simulink model "Hystersis_Relay_Logic"  (R2017a)
settings: Solver=FixedStepDiscrete  StartTime=0.0  StopTime=10.0  FixedStep=0.01  RelTol=1e-3
libraries: simulink x1, simulink_extras x1
settings Model: Creator=ACER  LastModifiedBy=peram
settings DataIOCC: ReturnWorkspaceOutputs=on
settings DebuggingCC: UnconnectedInputMsg=none  UnconnectedOutputMsg=none  UnconnectedLineMsg=none  SFMachineParentedDataDiag=error
settings ModelReferenceCC: EnableRefExpFcnMdlSchedulingChecks=off
settings SFSimCC: SimUseLocalCustomCode=on
settings RTWCC: RTWUseLocalCustomCode=on

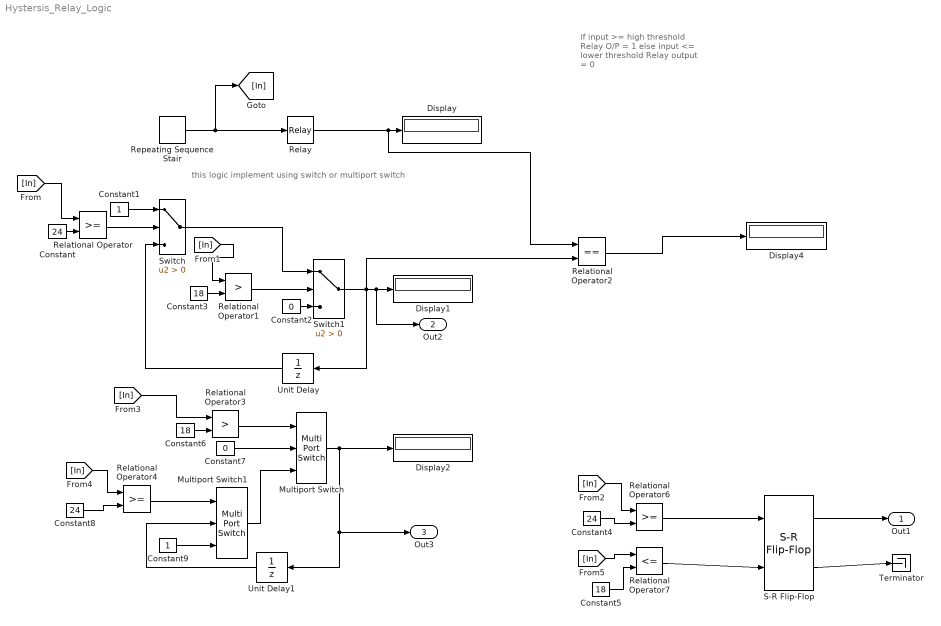
== system Hystersis_Relay_Logic ==
  note: if input >= high threshold
      | Relay O/P = 1
      | else
      | input <= lower threshold
      | Relay output = 0
  note: this logic implement using switch or multiport switch
  Constant : Constant  Value=24  OutDataTypeStr=Inherit: Inherit via back propagation
  Constant1 : Constant
  Constant2 : Constant  Value=0
  Constant3 : Constant  Value=18
  Constant4 : Constant  Value=24
  Constant5 : Constant  Value=18
  Constant6 : Constant  Value=18  OutDataTypeStr=Inherit: Inherit via back propagation
  Constant7 : Constant  Value=0  OutDataTypeStr=Inherit: Inherit via back propagation
  Constant8 : Constant  Value=24  OutDataTypeStr=Inherit: Inherit via back propagation
  Constant9 : Constant  OutDataTypeStr=Inherit: Inherit via back propagation
  Display{,1..2,4} (4 alike) : Display
  Multiport Switch : MultiPortSwitch  DataPortOrder=Zero-based contiguous  Inputs=2  OutDataTypeStr=Inherit: Inherit via back propagation
  Multiport Switch1 : MultiPortSwitch  DataPortOrder=Zero-based contiguous  Inputs=2  OutDataTypeStr=Inherit: Inherit via back propagation
  Relational Operator : RelationalOperator  OutDataTypeStr=boolean  RndMeth=Simplest
  Relational Operator1 : RelationalOperator  Operator=>  OutDataTypeStr=boolean  RndMeth=Simplest
  Relational Operator2 : RelationalOperator  Operator===  OutDataTypeStr=boolean  RndMeth=Simplest
  Relational Operator3 : RelationalOperator  Operator=>  OutDataTypeStr=boolean  RndMeth=Simplest
  Relational Operator4 : RelationalOperator  OutDataTypeStr=boolean  RndMeth=Simplest
  Relational Operator6 : RelationalOperator  OutDataTypeStr=boolean  RndMeth=Simplest
  Relational Operator7 : RelationalOperator  Operator=<=  OutDataTypeStr=boolean  RndMeth=Simplest
  Relay : Relay  OnSwitchValue=24  OffSwitchValue=18
  Repeating Sequence Stair : simulink/Sources/Repeating Sequence Stair  OutValues=[17 18 20 24 27 22 18 17 26 15].'  tsamp=-1  OutMin=[]  OutMax=[]  OutDataTypeStr=uint8  OutputDataTypeScalingMode=uint8  OutDataType=fixdt(0,8)  ConRadixGroup=Best Precision: Vector-wise  OutScaling=2^-12
  S-R Flip-Flop : simulink_extras/Flip Flops/S-R Flip-Flop  initial_condition=0
  Switch : Switch  Criteria=u2 > Threshold  OutDataTypeStr=Inherit: Inherit via back propagation
  Switch1 : Switch  Criteria=u2 > Threshold  OutDataTypeStr=Inherit: Inherit via back propagation
  Terminator : Terminator
  Unit Delay : UnitDelay  SampleTime=-1
  Unit Delay1 : UnitDelay  SampleTime=-1
  Out1 : Outport
  Out2 : Outport  Port=2  OutDataTypeStr=int8
  Out3 : Outport  Port=3  OutDataTypeStr=uint32
  wires:
  Relay/1 -> Relational Operator2/1, Display/1
  Repeating Sequence Stair/1 -> [In], Relay/1
  Relational Operator/1 -> Switch/2
  [In] -> Relational Operator/1
  Constant/1 -> Relational Operator/2
  Constant1/1 -> Switch/1
  Relational Operator1/1 -> Switch1/2
  [In] -> Relational Operator1/1
  Constant3/1 -> Relational Operator1/2
  Switch1/1 -> Relational Operator2/2, Unit Delay/1, Out2/1, Display1/1
  Unit Delay/1 -> Switch/3
  Constant6/1 -> Relational Operator3/2
  [In] -> Relational Operator3/1
  Relational Operator3/1 -> Multiport Switch/1
  Constant7/1 -> Multiport Switch/2
  Multiport Switch1/1 -> Multiport Switch/3
  [In] -> Relational Operator4/1
  Constant8/1 -> Relational Operator4/2
  Relational Operator4/1 -> Multiport Switch1/1
  Constant9/1 -> Multiport Switch1/3
  Constant2/1 -> Switch1/3
  Switch/1 -> Switch1/1
  Multiport Switch/1 -> Display2/1, Out3/1, Unit Delay1/1
  Unit Delay1/1 -> Multiport Switch1/2
  Relational Operator2/1 -> Display4/1
  [In] -> Relational Operator6/1
  Constant4/1 -> Relational Operator6/2
  [In] -> Relational Operator7/1
  Constant5/1 -> Relational Operator7/2
  Relational Operator7/1 -> S-R Flip-Flop/2
  Relational Operator6/1 -> S-R Flip-Flop/1
  S-R Flip-Flop/1 -> Out1/1
  S-R Flip-Flop/2 -> Terminator/1
